simulink model "sortie_photorecepteurs"  (R2020a)
settings: Solver=VariableStepAuto  StartTime=0.0  StopTime=10.0  RelTol=1e-3
libraries: simulink x1
settings Model: Creator=omsso  LastModifiedBy=omsso

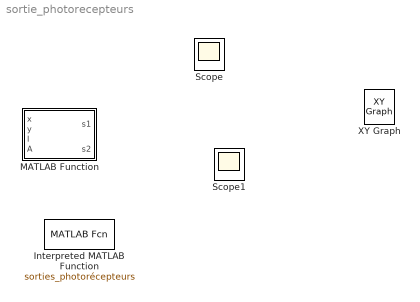
== system sortie_photorecepteurs ==
  Interpreted MATLAB Function : MATLABFcn  MATLABFcn=sorties_photorécepteurs
  MATLAB Function : MATLAB Function  TreatAsAtomicUnit=on
  Scope : Scope
  Scope1 : Scope
  XY Graph : simulink/Sinks/XY Graph  xmin=-1  xmax=1  ymin=-1  ymax=1  st=-1

== matlab function sortie_photorecepteurs/MATLAB Function ==
  data: x input; s1 output; y input; I input; A input; s2 output
function [s1,s2]= sortie_photorecepteurs(x,y, I,A)

deltarho =3.8;
deltaphi= deltarho;
thetas=zeros(100);

for i=1:(size(I,1))
    thetas(i)=atan2(-y,I(i,1)-x)*180/pi;
end

v1= find((-90+deltarho/2-1.3*deltarho<=thetas)&(thetas<=-90+deltaphi/2+1.3*deltarho));
v2=find((-90-deltarho/2-1.3*deltarho<=thetas)&(thetas<=-90-deltaphi/2+1.3*deltarho))
 %angle à partir duquel ph 1 perçoit

                             
s1=0;                         
s2=0;                         
ph1=0;
ph2=0;
theta1=thetas(v1);
theta2=thetas(v2);
N=length(v2);
thetaMax=9,88;
%photorécepteur1: ajouter les bords + recalibrage
for i=1:(N-1)
    theta1=(abs(thetas(v2(i)-(-90-deltaphi/2-1.3*deltaphi)))/thetaMax*1976;
    theta2=(abs(thetas(v2(i+1)-(-90-deltaphi/2-1.3*deltaphi)))/thetaMax*1976;
    ph1= ph1+I(v2(i),2)*A(floor(theta2),floor(theta1));
end

%photorécepteur2
for i=1:(length(v1)-1)
    theta1=abs(thetas(v1(i)-(-90+deltaphi/2-1.3*deltaphi))/thetaMax*1976
    theta2=abs(thetas(v1(i+1)-(-90+deltaphi/2-1.3*deltaphi))/thetaMax*1976;
    ph2=ph2+I(v1(i),2)*A(floor(theta1),floor(theta2));
end
s1=ph1;
s2=ph2;
end
